simulink model "BMD_2_backup"  (R2025b)
settings: Solver=FixedStepAuto  StartTime=0.0  StopTime=15  FixedStep=0.005  RelTol=1e-3
values from neighbouring files (symbols this model uses):
  FPV_mass = 0.8    [Soft.m]
  g = 9.81    [Soft.m]
  ks = 0    [Soft.m]
  p_0 = 1013.25    [Soft.m]
  Q2Ts = forcetomotors()    [Soft.m]    (also in forcetomotors.m = inv(Ts2Q))
  takeOffDuration = 2    [Soft.m]
  Ts = 0.005    [Soft.m]
undefined symbols (not defined in the file or in its folder): CdA, DiscIntNeverNeededParam, Dw, kd_dz, kd_pos_dx, kd_pos_dy, kd_pq, kd_pr, kd_y, kd_z, ki_dz, ki_pos_dx, ki_pos_dy, ki_pq, ki_pr, ki_y, ki_z, kp_dz, kp_pos_dx, kp_pos_dy, kp_pos_x, kp_pos_y, kp_pq, kp_pr, kp_y, kp_z, pInitialization, rho
libraries: simulink x43, discretizing x18, slpidlib x3, SignalEditorBlockLib x2, shared6dof x1, dynamicsLibrary x1, aerolibasang x1, aerolibnav x1
(part 7 of 22)

== system BMD_2_backup/FCS/Controller/tau_contorller ==
  Yaw_ref [rad/s] : Inport
  In2 : Inport  Port=2
  r_s : Inport  Port=3
  In4 : Inport  Port=4
  Compare To Constant : simulink/Logic and Bit Operations/Compare To Constant  relop===  const=0.00  OutDataTypeStr=boolean
  Constant1 : Constant  Value=0
  Discrete-Time Integrator : DiscreteIntegrator  gainval=0.05  SampleTime=-1  ICPrevOutput=DiscIntNeverNeededParam  ICPrevScaledInput=DiscIntNeverNeededParam
  Gain1 : Gain  Gain=0.8
  Gain_yaw_in : Gain  Gain=1.3
  NOT : Logic  Operator=NOT  IconShape=distinctive  AllPortsSameDT=off  OutDataTypeStr=boolean
  PID Controller (2DOF) : slpidlib/PID Controller (2DOF)  Controller=PID  Form=Parallel  TimeDomain=Discrete-time  UseExternalTs=off  SampleTime=0.005  IntegratorMethod=Forward Euler  FilterMethod=Forward Euler  ControllerParametersSource=internal  P=kp_y  I=ki_y  UseKiTs=off  D=kd_y  UseExternalDerivativeSource=off  N=100  UseFilter=on  b=1  c=0  TunerSelectOption=Transfer Function Based (PID Tuner App)  InitialConditionSource=internal  InitialConditionForIntegrator=0  InitialConditionForFilter=0  DifferentiatorICPrevScaledInput=0  ExternalReset=none  TrackingMode=off  Kt=1  LimitOutput=off  SatLimitsSource=internal  UpperSaturationLimit=inf  LowerSaturationLimit=-inf  LinearizeAsGain=on  AntiWindupMode=none  Kb=1  LimitIntegrator=on  UpperIntegratorSaturationLimit=0.02  LowerIntegratorSaturationLimit=-0.02  POutMin=[]  POutMax=[]  IOutMin=[]  IOutMax=[]  DOutMin=[]  DOutMax=[]  NOutMin=[]  NOutMax=[]  bOutMin=[]  bOutMax=[]  cOutMin=[]  cOutMax=[]  SumOutMin=[]  SumOutMax=[]  SaturationOutMin=[]  SaturationOutMax=[]  PParamMin=[]  PParamMax=[]  IParamMin=[]  IParamMax=[]  DParamMin=[]  DParamMax=[]  NParamMin=[]  NParamMax=[]  bParamMin=[]  bParamMax=[]  cParamMin=[]  cParamMax=[]  KbParamMin=[]  KbParamMax=[]  KtParamMin=[]  KtParamMax=[]  KbOutMin=[]  KbOutMax=[]  KtOutMin=[]  KtOutMax=[]  IntegratorOutMin=[]  IntegratorOutMax=[]  FilterOutMin=[]  FilterOutMax=[]  SumI1OutMin=[]  SumI1OutMax=[]  SumI2OutMin=[]  SumI2OutMax=[]  SumI3OutMin=[]  SumI3OutMax=[]  SumI4OutMin=[]  SumI4OutMax=[]  SumDOutMin=[]  SumDOutMax=[]  Sum1OutMin=[]  Sum1OutMax=[]  Sum2OutMin=[]  Sum2OutMax=[]  Sum3OutMin=[]  Sum3OutMax=[]  DifferentiatorOutMin=[]  DifferentiatorOutMax=[]  FilterDiffOutCoefMin=[]  FilterDiffOutCoefMax=[]  ReciprocalOutMin=[]  ReciprocalOutMax=[]  SumDenOutMin=[]  SumDenOutMax=[]  SumNumOutMin=[]  SumNumOutMax=[]  DivideOutMin=[]  DivideOutMax=[]  UdiffTsProdOutMin=[]  UdiffTsProdOutMax=[]  NTsProdOutMin=[]  NTsProdOutMax=[]  UintegralTsProdOutMin=[]  UintegralTsProdOutMax=[]  UngainTsProdOutMin=[]  UngainTsProdOutMax=[]  ClampingZeroOutDataTypeStr=Inherit: Inherit via back propagation  ClampingZeroOutMin=[]  ClampingZeroOutMax=[]  FilterDenConstantOutDataTypeStr=Inherit: Inherit via back propagation  FilterDenConstantOutMin=[]  FilterDenConstantOutMax=[]  PCopyOutDataTypeStr=Inherit: Inherit via back propagation  PCopyOutMin=[]  PCopyOutMax=[]  NCopyOutDataTypeStr=Inherit: Inherit via back propagation  NCopyOutMin=[]  NCopyOutMax=[]  IntegratorContinuousStateAttributes=''  IntegratorStateMustResolveToSignalObject=off  IntegratorRTWStateStorageClass=Auto  FilterContinuousStateAttributes=''  FilterStateMustResolveToSignalObject=off  FilterRTWStateStorageClass=Auto  ParallelPVariant=InternalParameters  IdealPVariant=Disabled  IVariant=InternalParameters  DVariant=InternalParameters  bVariant=InternalParameters  cVariant=InternalParameters  IntegratorVariant=Discrete  SatVariant=Disabled  AWVariant=Passthrough  PCopyVariant=Disabled  TRVariant=Disabled  FdbkBlocksVariant=Forward  IdealPFdbkVariant=Disabled  SatFdbkVariant=Disabled  DerivativeFilterVariant=ForwardEulerFilter  NVariant=InternalParameters  NCopyVariant=Disabled  FilterICVariant=InternalICsFilter  IntegratorICVariant=InternalICs  ExternalResetVariant=Disabled  TRSumVariant=Passthrough  SumFdbkVariant=Disabled  SumVariant=Sum_PID  TsampFilterVariant=InternalTs  TsampNgainVariant=Passthrough  TsampIntegralVariant=Disabled_SignalSpec  ExternalSaturationOutDataTypeStr=Inherit: Same as second input  DerivativeSourceVariant=ErrorSignal  PreIntVariant=InternalPreInt
  Rate Limiter1 : RateLimiter  RisingSlewLimit=2.0  FallingSlewLimit=-2.0  SampleTimeMode=inherited
  Saturation : Saturate  LinearizeAsGain=off
  Saturation_yaw_out : Saturate  UpperLimit=05  OutDataTypeStr=double
  Scope : Scope
      settings: ActiveDisplayYMinimum=-1  ActiveDisplayYMaximum=1  DataLoggingVariableName=ScopeData36
  Scope2 : Scope
      settings: ActiveDisplayYMinimum=-0.021957566607169628  ActiveDisplayYMaximum=0.19761914569671202  DataLoggingVariableName=ScopeData40
  Sum : Sum  Inputs=|+-
  Sum1 : Sum  Inputs=|++
  Switch1 : Switch  Criteria=u2 > Threshold  OutDataTypeStr=single  SaturateOnIntegerOverflow=off  InputSameDT=off
  Switch2 : Switch  Criteria=u2 > Threshold  OutDataTypeStr=single  SaturateOnIntegerOverflow=off  InputSameDT=off
  Switch3 : Switch  Criteria=u2 > Threshold  OutDataTypeStr=single  SaturateOnIntegerOverflow=off  InputSameDT=off
  Terminator : Terminator
  Unit Delay : UnitDelay  SampleTime=-1  HasFrameUpgradeWarning=on
  tau_yaw : Outport
  wires:
  Discrete-Time Integrator/1 -> Scope/1
  Constant1/1 -> Switch1/1
  Yaw_ref [rad/s]/1 -> Compare To Constant/1, Switch1/3
  Rate Limiter1/1 -> Gain_yaw_in/1
  Saturation_yaw_out/1 -> tau_yaw/1
  Switch1/1 -> Rate Limiter1/1
  In2/1 -> Terminator/1
  PID Controller (2DOF)/1 -> Saturation_yaw_out/1
  Compare To Constant/1 -> Switch2/2, NOT/1, Switch1/2
  In4/1 -> Sum/2, Switch2/3
  Switch2/1 -> Unit Delay/1, Scope2/1, Sum/1
  Unit Delay/1 -> Switch2/1
  Sum/1 -> Gain1/1
  Gain1/1 -> Sum1/2
  Sum1/1 -> Saturation/1
  NOT/1 -> Switch3/2
  Gain_yaw_in/1 -> Switch3/1
  Switch3/1 -> PID Controller (2DOF)/1
  Saturation/1 -> Switch3/3
  r_s/1 -> Discrete-Time Integrator/1, PID Controller (2DOF)/2

== system BMD_2_backup/FCS/filters/Subsystem ==
  GPS_s : Inport
  pressure_f : Inport  Port=2
  ax,ay,ax_f : Inport  Port=3
  orient_earth : Inport  Port=4
  Data Type Conversion3 : DataTypeConversion  OutDataTypeStr=single  SaturateOnIntegerOverflow=off  RndMeth=Floor
  Scope : Scope  NumInputPorts=2
      settings: ActiveDisplayYMinimum=-1.9435508120805021  ActiveDisplayYMaximum=15.792740793898702  DataLoggingVariableName=ScopeData52
  Scope1 : Scope
      settings: ActiveDisplayYMinimum=-1  ActiveDisplayYMaximum=1  DataLoggingVariableName=ScopeData55
  body2earth : Subsystem
  x,y,z,dy,dy,dz : Subsystem
  x,y,z : Outport
  dx,dy,dz : Outport  Port=2
  wires:
  x,y,z,dy,dy,dz/2(dx,dy,dz) -> Scope1/1, dx,dy,dz/1
  body2earth/1(Out1) -> x,y,z,dy,dy,dz/1(ax,ay,az_earth)  "ax,ay,az_earth"
  orient_earth/1 -> Data Type Conversion3/1
  ax,ay,ax_f/1 -> body2earth/1(ax,ay,az)
  x,y,z,dy,dy,dz/1(x,y,z) -> Scope/1, x,y,z/1
  pressure_f/1 -> x,y,z,dy,dy,dz/2(pressure_f)
  Data Type Conversion3/1 -> body2earth/2(orient_f)
  GPS_s/1 -> x,y,z,dy,dy,dz/3(GPS_s)

== system BMD_2_backup/FCS/filters/Subsystem1 ==
  ax,ay,ax_f : Inport
  p,q,r_f : Inport  Port=2
  Demux2 : Demux  Outputs=3
  Mux1 : Mux  Inputs=3
  pitch_kalman : Subsystem
  roll_kalman : Subsystem
  yaw_filter : Subsystem
  orient_earth : Outport
  wires:
  Mux1/1 -> orient_earth/1  "orient_earth"
  Demux2/3 -> yaw_filter/1(In1)  "r"
  Demux2/2 -> pitch_kalman/2(pitch)  "q"
  ax,ay,ax_f/1 -> roll_kalman/1(ax,ay,az), pitch_kalman/1(ax,ay,az)
  Demux2/1 -> roll_kalman/2(p)  "p"
  pitch_kalman/1(Out1) -> Mux1/2  "pitch_f"
  p,q,r_f/1 -> Demux2/1
  yaw_filter/1(Out1) -> Mux1/3  "yaw_f"
  roll_kalman/1(roll_f) -> Mux1/1  "roll_f"

== system BMD_2_backup/FCS/filters/pqr_LPF1 ==
  1 : Inport
  Demux : Demux  Outputs=3
  Mux : Mux  Inputs=3
  Transfer Fcn1 : discretizing/Discretized Transfer Fcn  Numerator=[1]  Denominator=[0.15 1]  AbsTol=auto  SampleTime=0.005  method=zoh  Wc=0
  Transfer Fcn2 : discretizing/Discretized Transfer Fcn  Numerator=[1]  Denominator=[0.15 1]  AbsTol=auto  SampleTime=0.005  method=zoh  Wc=0
  Transfer Fcn3 : discretizing/Discretized Transfer Fcn  Numerator=[1]  Denominator=[0.15 1]  AbsTol=auto  SampleTime=0.005  method=zoh  Wc=0
  ax,ay,az : Outport
  wires:
  1/1 -> Demux/1
  Mux/1 -> ax,ay,az/1
  Demux/1 -> Transfer Fcn3/1
  Demux/2 -> Transfer Fcn1/1
  Demux/3 -> Transfer Fcn2/1
  Transfer Fcn3/1 -> Mux/1
  Transfer Fcn2/1 -> Mux/3
  Transfer Fcn1/1 -> Mux/2

== system BMD_2_backup/FCS/filters/pqr_LPF2 ==
  p,q,r : Inport
  Demux : Demux  Outputs=3
  Mux : Mux  Inputs=3
  Transfer Fcn1 : discretizing/Discretized Transfer Fcn  Numerator=[1]  Denominator=[0.15 1]  AbsTol=auto  SampleTime=0.005  method=zoh  Wc=0
  Transfer Fcn2 : discretizing/Discretized Transfer Fcn  Numerator=[1]  Denominator=[0.15 1]  AbsTol=auto  SampleTime=0.005  method=zoh  Wc=0
  Transfer Fcn3 : discretizing/Discretized Transfer Fcn  Numerator=[1]  Denominator=[0.15 1]  AbsTol=auto  SampleTime=0.005  method=zoh  Wc=0
  p,q,r_f : Outport
  wires:
  p,q,r/1 -> Demux/1
  Mux/1 -> p,q,r_f/1
  Demux/1 -> Transfer Fcn3/1
  Demux/2 -> Transfer Fcn1/1
  Demux/3 -> Transfer Fcn2/1
  Transfer Fcn2/1 -> Mux/3  "temp_f"
  Transfer Fcn3/1 -> Mux/1  "temp_f"
  Transfer Fcn1/1 -> Mux/2  "temp_f"

== system BMD_2_backup/Model/Subsystem/Motor Forces and Torques ==
  Vb : Inport
  Density : Inport  Port=2
  pqr : Inport  Port=3
  Motor Commands : Inport  Port=4
  D1 : Constant  Value=0.044
  D2 : Constant  Value=0.044
  D3 : Constant  Value=-0.044
  D4 : Constant  Value=-0.044
  For Each Subsystem : Subsystem  TreatAsAtomicUnit=on
  Gain : Gain  Gain=[0.0030015 0.0030015 0.0030015 0.0030015]
  MotorsToW : Subsystem
  Sum of Elements : Sum  Inputs=+  CollapseMode=Specified dimension  CollapseDim=2
  Sum of Elements1 : Sum  Inputs=+  CollapseMode=Specified dimension  CollapseDim=2
  Vector Concatenate : Concatenate  NumInputs=4  Mode=Multidimensional array  ConcatenateDimension=2
  Motor Forces : Outport  Unit=N  VectorParamsAs1DForOutWhenUnconnected=off
  Motor Torques : Outport  Port=2  Unit=N*m  VectorParamsAs1DForOutWhenUnconnected=off
  wires:
  D4/1 -> Vector Concatenate/4
  Vector Concatenate/1 -> For Each Subsystem/5(D)
  For Each Subsystem/2(Moments) -> Sum of Elements1/1
  pqr/1 -> For Each Subsystem/3(Omega)
  Vb/1 -> For Each Subsystem/1(Vb)
  D1/1 -> Vector Concatenate/1
  D3/1 -> Vector Concatenate/3
  D2/1 -> Vector Concatenate/2
  Sum of Elements1/1 -> Motor Torques/1
  Density/1 -> For Each Subsystem/2(rho)
  Sum of Elements/1 -> Motor Forces/1
  For Each Subsystem/1(Forces) -> Sum of Elements/1
  Motor Commands/1 -> Gain/1
  Gain/1 -> For Each Subsystem/4(w)

== system BMD_2_backup/Model/Subsystem/drag forces ==
  pressure : Inport
  V_b : Inport  Port=2
  Dynamic Pressure : aerolibasang/Dynamic Pressure
  Out1 : Outport
  wires:
  Dynamic Pressure/1 -> Out1/1
  V_b/1 -> Dynamic Pressure/1
  pressure/1 -> Dynamic Pressure/2

== system BMD_2_backup/Model/Subsystem/gravity forces ==
  gravity : Inport
  DCM(angeles) : Inport  Port=2
  Display : Display
  Gain : Gain  Gain=FPV_mass
  Matrix Multiply : Product  Multiplication=Matrix(*)
  Scope : Scope
      settings: ActiveDisplayYMinimum=-0.613125221623891  ActiveDisplayYMaximum=5.5181252577452655  DataLoggingVariableName=ScopeData70
  Out1 : Outport
  wires:
  gravity/1 -> Gain/1
  Gain/1 -> Matrix Multiply/2
  Matrix Multiply/1 -> Display/1, Scope/1, Out1/1
  DCM(angeles)/1 -> Matrix Multiply/1

== system BMD_2_backup/Sensors/Subsystem/Subsystem ==
  Mux : Mux  Inputs=3
  Zero1 : Constant  Value=0  OutDataTypeStr=single
  Zero2 : Constant  Value=0  OutDataTypeStr=single
  Zero3 : Constant  Value=0  OutDataTypeStr=single
  Out1 : Outport
  wires:
  Zero2/1 -> Mux/1
  Zero1/1 -> Mux/2
  Zero3/1 -> Mux/3
  Mux/1 -> Out1/1

== system BMD_2_backup/Sensors/Subsystem1/Subsystem ==
  Mux : Mux  Inputs=3
  Zero1 : Constant  Value=0  OutDataTypeStr=single
  Zero2 : Constant  Value=0  OutDataTypeStr=single
  Zero3 : Constant  Value=0  OutDataTypeStr=single
  Out1 : Outport
  wires:
  Zero2/1 -> Mux/1
  Zero1/1 -> Mux/2
  Zero3/1 -> Mux/3
  Mux/1 -> Out1/1

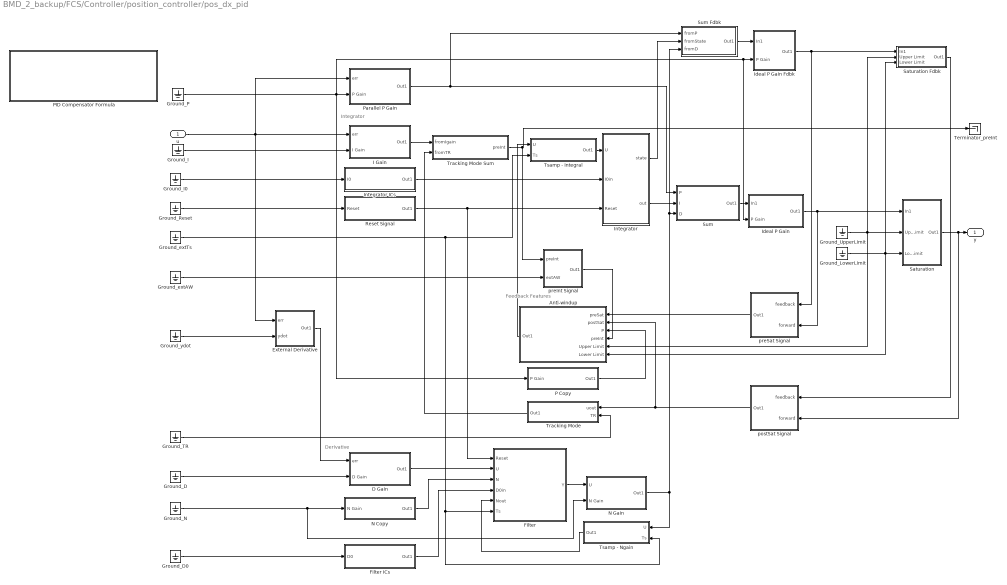
== system BMD_2_backup/FCS/Controller/position_controller/pos_dx_pid ==
  note: Feedback Features
  note: Derivative
  note: Integrator
  u : Inport  SampleTime=SampleTime
  Anti-windup : Subsystem  Variant=on  VariantControlMode=label  VariantControl=Variant1  LabelModeActiveChoice=Passthrough
  D Gain : Subsystem  Variant=on  VariantControlMode=label  VariantControl=Variant1  LabelModeActiveChoice=InternalParameters
  External Derivative : Subsystem  Variant=on  VariantControlMode=label  VariantControl=Variant1  LabelModeActiveChoice=ErrorSignal
  Filter : Subsystem  Variant=on  VariantControlMode=label  LabelModeActiveChoice=ForwardEulerFilter
  Filter ICs : Subsystem  Variant=on  VariantControlMode=label  VariantControl=Variant1  LabelModeActiveChoice=InternalICsFilter
  Ground_D : Ground
  Ground_D0 : Ground
  Ground_I : Ground
  Ground_I0 : Ground
  Ground_LowerLimit : Ground
  Ground_N : Ground
  Ground_P : Ground
  Ground_Reset : Ground
  Ground_TR : Ground  DisableCoverage=on
  Ground_UpperLimit : Ground
  Ground_extAW : Ground
  Ground_extTs : Ground
  Ground_ydot : Ground
  I Gain : Subsystem  Variant=on  VariantControlMode=label  VariantControl=Variant1  LabelModeActiveChoice=InternalParameters
  Ideal P Gain : Subsystem  Variant=on  VariantControlMode=label  VariantControl=Variant1  LabelModeActiveChoice=Disabled
  Ideal P Gain Fdbk : Subsystem  Variant=on  VariantControlMode=label  VariantControl=Variant1  LabelModeActiveChoice=Disabled
  Integrator : Subsystem  Variant=on  VariantControlMode=label  LabelModeActiveChoice=Discrete
  Integrator ICs : Subsystem  Variant=on  VariantControlMode=label  VariantControl=Variant1  LabelModeActiveChoice=InternalICs
  N Copy : Subsystem  Variant=on  VariantControlMode=label  LabelModeActiveChoice=Disabled
  N Gain : Subsystem  Variant=on  VariantControlMode=label  VariantControl=Variant1  LabelModeActiveChoice=InternalParameters
  P Copy : Subsystem  Variant=on  VariantControlMode=label  LabelModeActiveChoice=Disabled
  PID Compensator Formula : Subsystem
      mask Display: image('C:\Program Files\MATLAB\R2025b\toolbox\simulink\library\pid\pid_Images\PID_Parallel_DT_00.png','center');
  Parallel P Gain : Subsystem  Variant=on  VariantControlMode=label  VariantControl=Variant1  LabelModeActiveChoice=InternalParameters
  Reset Signal : Subsystem  Variant=on  VariantControlMode=label  VariantControl=Variant1  LabelModeActiveChoice=Disabled
  Saturation : Subsystem  Variant=on  VariantControlMode=label  LabelModeActiveChoice=Enabled
  Saturation Fdbk : Subsystem  Variant=on  VariantControlMode=label  LabelModeActiveChoice=Disabled
  Sum : Subsystem  Variant=on  VariantControlMode=label  LabelModeActiveChoice=Sum_PID
  Sum Fdbk : Subsystem  DisableCoverage=on  Variant=on  VariantControlMode=label  LabelModeActiveChoice=Disabled
  Terminator_preInt : Terminator
  Tracking Mode : Subsystem  Variant=on  VariantControlMode=label  VariantControl=Variant1  LabelModeActiveChoice=Disabled
  Tracking Mode Sum : Subsystem  Variant=on  VariantControlMode=label  LabelModeActiveChoice=Passthrough
  Tsamp - Integral : Subsystem  Variant=on  VariantControlMode=label  LabelModeActiveChoice=Disabled_SignalSpec
  Tsamp - Ngain : Subsystem  Variant=on  VariantControlMode=label  LabelModeActiveChoice=Passthrough
  postSat Signal : Subsystem  Variant=on  VariantControlMode=label  VariantControl=Variant1  LabelModeActiveChoice=Forward
  preInt Signal : Subsystem  Variant=on  VariantControlMode=label  VariantControl=Variant1  LabelModeActiveChoice=InternalPreInt
  preSat Signal : Subsystem  Variant=on  VariantControlMode=label  VariantControl=Variant1  LabelModeActiveChoice=Forward
  y : Outport  SampleTime=SampleTime
  wires:
  Ground_extAW/1 -> preInt Signal/2(extAW)
  preInt Signal/1(Out1) -> Anti-windup/4(preInt)
  External Derivative/1(Out1) -> D Gain/1(err)
  Ground_ydot/1 -> External Derivative/2(ydot)
  Ground_LowerLimit/1 -> Saturation/3(Lower Limit), Anti-windup/6(Lower Limit), Saturation Fdbk/3(Lower Limit)
  Ground_UpperLimit/1 -> Saturation/2(Upper Limit), Saturation Fdbk/2(Upper Limit), Anti-windup/5(Upper Limit)
  Tsamp - Ngain/1(Out1) -> Filter/5(Nout)
  Anti-windup/1(Out1) -> Tsamp - Integral/1(U)
  Ground_extTs/1 -> Tsamp - Integral/2(Ts), Filter/6(Ts), Tsamp - Ngain/2(Ts)
  Tsamp - Integral/1(Out1) -> Integrator/1(U)
  Tracking Mode/1(Out1) -> Tracking Mode Sum/2(fromTR)
  Ground_I0/1 -> Integrator ICs/1(I0)
  Filter ICs/1(Out1) -> Filter/4(D0in)
  N Copy/1(Out1) -> Filter/3(N)
  D Gain/1(Out1) -> Filter/2(U)
  Ground_D0/1 -> Filter ICs/1(D0)
  Ground_Reset/1 -> Reset Signal/1(Reset)
  N Gain/1(Out1) -> Tsamp - Ngain/1(U), Sum/3(D), Sum Fdbk/3(fromD)
  postSat Signal/1(Out1) -> Anti-windup/2(postSat), Tracking Mode/1(uout)
  preSat Signal/1(Out1) -> Anti-windup/1(preSat)
  Saturation Fdbk/1(Out1) -> postSat Signal/1(feedback)
  P Copy/1(Out1) -> Anti-windup/3(P)
  Ground_TR/1 -> Tracking Mode/2(TR)
  Ground_N/1 -> N Copy/1(N Gain), N Gain/2(N Gain)
  Ideal P Gain Fdbk/1(Out1) -> preSat Signal/1(feedback), Saturation Fdbk/1(In1)
  Sum Fdbk/1(Out1) -> Ideal P Gain Fdbk/1(In1)
  I Gain/1(Out1) -> Tracking Mode Sum/1(fromIgain)
  Saturation/1(Out1) -> y/1, postSat Signal/2(forward)
  Filter/1(Y) -> N Gain/1(U)
  Ground_D/1 -> D Gain/2(D Gain)
  Ideal P Gain/1(Out1) -> Saturation/1(In1), preSat Signal/2(forward)
  u/1 -> External Derivative/1(err), Parallel P Gain/1(err), I Gain/1(err)
  Parallel P Gain/1(Out1) -> Sum/1(P), Sum Fdbk/1(fromP)
  Sum/1(Out1) -> Ideal P Gain/1(In1)
  Ground_P/1 -> Ideal P Gain Fdbk/2(P Gain), Ideal P Gain/2(P Gain), Parallel P Gain/2(P Gain), P Copy/1(P Gain)
  Tracking Mode Sum/1(preInt) -> Terminator_preInt/1, preInt Signal/1(preInt)
  Ground_I/1 -> I Gain/2(I Gain)
  Integrator ICs/1(Out1) -> Integrator/2(I0in)
  Integrator/2(out) -> Sum/2(I)
  Integrator/1(state) -> Sum Fdbk/2(fromState)
  Reset Signal/1(Out1) -> Filter/1(Reset), Integrator/3(Reset)

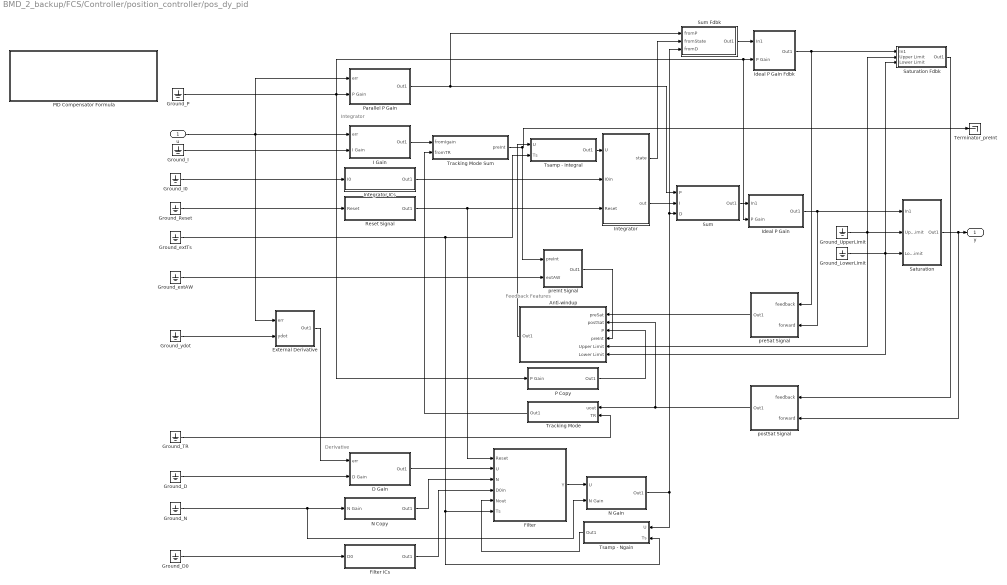
== system BMD_2_backup/FCS/Controller/position_controller/pos_dy_pid ==
  note: Feedback Features
  note: Derivative
  note: Integrator
  u : Inport  SampleTime=SampleTime
  Anti-windup : Subsystem  Variant=on  VariantControlMode=label  VariantControl=Variant1  LabelModeActiveChoice=Passthrough
  D Gain : Subsystem  Variant=on  VariantControlMode=label  VariantControl=Variant1  LabelModeActiveChoice=InternalParameters
  External Derivative : Subsystem  Variant=on  VariantControlMode=label  VariantControl=Variant1  LabelModeActiveChoice=ErrorSignal
  Filter : Subsystem  Variant=on  VariantControlMode=label  LabelModeActiveChoice=ForwardEulerFilter
  Filter ICs : Subsystem  Variant=on  VariantControlMode=label  VariantControl=Variant1  LabelModeActiveChoice=InternalICsFilter
  Ground_D : Ground
  Ground_D0 : Ground
  Ground_I : Ground
  Ground_I0 : Ground
  Ground_LowerLimit : Ground
  Ground_N : Ground
  Ground_P : Ground
  Ground_Reset : Ground
  Ground_TR : Ground  DisableCoverage=on
  Ground_UpperLimit : Ground
  Ground_extAW : Ground
  Ground_extTs : Ground
  Ground_ydot : Ground
  I Gain : Subsystem  Variant=on  VariantControlMode=label  VariantControl=Variant1  LabelModeActiveChoice=InternalParameters
  Ideal P Gain : Subsystem  Variant=on  VariantControlMode=label  VariantControl=Variant1  LabelModeActiveChoice=Disabled
  Ideal P Gain Fdbk : Subsystem  Variant=on  VariantControlMode=label  VariantControl=Variant1  LabelModeActiveChoice=Disabled
  Integrator : Subsystem  Variant=on  VariantControlMode=label  LabelModeActiveChoice=Discrete
  Integrator ICs : Subsystem  Variant=on  VariantControlMode=label  VariantControl=Variant1  LabelModeActiveChoice=InternalICs
  N Copy : Subsystem  Variant=on  VariantControlMode=label  LabelModeActiveChoice=Disabled
  N Gain : Subsystem  Variant=on  VariantControlMode=label  VariantControl=Variant1  LabelModeActiveChoice=InternalParameters
  P Copy : Subsystem  Variant=on  VariantControlMode=label  LabelModeActiveChoice=Disabled
  PID Compensator Formula : Subsystem
      mask Display: image('C:\Program Files\MATLAB\R2025b\toolbox\simulink\library\pid\pid_Images\PID_Parallel_DT_00.png','center');
  Parallel P Gain : Subsystem  Variant=on  VariantControlMode=label  VariantControl=Variant1  LabelModeActiveChoice=InternalParameters
  Reset Signal : Subsystem  Variant=on  VariantControlMode=label  VariantControl=Variant1  LabelModeActiveChoice=Disabled
  Saturation : Subsystem  Variant=on  VariantControlMode=label  LabelModeActiveChoice=Enabled
  Saturation Fdbk : Subsystem  Variant=on  VariantControlMode=label  LabelModeActiveChoice=Disabled
  Sum : Subsystem  Variant=on  VariantControlMode=label  LabelModeActiveChoice=Sum_PID
  Sum Fdbk : Subsystem  DisableCoverage=on  Variant=on  VariantControlMode=label  LabelModeActiveChoice=Disabled
  Terminator_preInt : Terminator
  Tracking Mode : Subsystem  Variant=on  VariantControlMode=label  VariantControl=Variant1  LabelModeActiveChoice=Disabled
  Tracking Mode Sum : Subsystem  Variant=on  VariantControlMode=label  LabelModeActiveChoice=Passthrough
  Tsamp - Integral : Subsystem  Variant=on  VariantControlMode=label  LabelModeActiveChoice=Disabled_SignalSpec
  Tsamp - Ngain : Subsystem  Variant=on  VariantControlMode=label  LabelModeActiveChoice=Passthrough
  postSat Signal : Subsystem  Variant=on  VariantControlMode=label  VariantControl=Variant1  LabelModeActiveChoice=Forward
  preInt Signal : Subsystem  Variant=on  VariantControlMode=label  VariantControl=Variant1  LabelModeActiveChoice=InternalPreInt
  preSat Signal : Subsystem  Variant=on  VariantControlMode=label  VariantControl=Variant1  LabelModeActiveChoice=Forward
  y : Outport  SampleTime=SampleTime
  wires:
  Ground_extAW/1 -> preInt Signal/2(extAW)
  preInt Signal/1(Out1) -> Anti-windup/4(preInt)
  External Derivative/1(Out1) -> D Gain/1(err)
  Ground_ydot/1 -> External Derivative/2(ydot)
  Ground_LowerLimit/1 -> Saturation/3(Lower Limit), Anti-windup/6(Lower Limit), Saturation Fdbk/3(Lower Limit)
  Ground_UpperLimit/1 -> Saturation/2(Upper Limit), Saturation Fdbk/2(Upper Limit), Anti-windup/5(Upper Limit)
  Tsamp - Ngain/1(Out1) -> Filter/5(Nout)
  Anti-windup/1(Out1) -> Tsamp - Integral/1(U)
  Ground_extTs/1 -> Tsamp - Integral/2(Ts), Filter/6(Ts), Tsamp - Ngain/2(Ts)
  Tsamp - Integral/1(Out1) -> Integrator/1(U)
  Tracking Mode/1(Out1) -> Tracking Mode Sum/2(fromTR)
  Ground_I0/1 -> Integrator ICs/1(I0)
  Filter ICs/1(Out1) -> Filter/4(D0in)
  N Copy/1(Out1) -> Filter/3(N)
  D Gain/1(Out1) -> Filter/2(U)
  Ground_D0/1 -> Filter ICs/1(D0)
  Ground_Reset/1 -> Reset Signal/1(Reset)
  N Gain/1(Out1) -> Tsamp - Ngain/1(U), Sum/3(D), Sum Fdbk/3(fromD)
  postSat Signal/1(Out1) -> Anti-windup/2(postSat), Tracking Mode/1(uout)
  preSat Signal/1(Out1) -> Anti-windup/1(preSat)
  Saturation Fdbk/1(Out1) -> postSat Signal/1(feedback)
  P Copy/1(Out1) -> Anti-windup/3(P)
  Ground_TR/1 -> Tracking Mode/2(TR)
  Ground_N/1 -> N Copy/1(N Gain), N Gain/2(N Gain)
  Ideal P Gain Fdbk/1(Out1) -> preSat Signal/1(feedback), Saturation Fdbk/1(In1)
  Sum Fdbk/1(Out1) -> Ideal P Gain Fdbk/1(In1)
  I Gain/1(Out1) -> Tracking Mode Sum/1(fromIgain)
  Saturation/1(Out1) -> y/1, postSat Signal/2(forward)
  Filter/1(Y) -> N Gain/1(U)
  Ground_D/1 -> D Gain/2(D Gain)
  Ideal P Gain/1(Out1) -> Saturation/1(In1), preSat Signal/2(forward)
  u/1 -> External Derivative/1(err), Parallel P Gain/1(err), I Gain/1(err)
  Parallel P Gain/1(Out1) -> Sum/1(P), Sum Fdbk/1(fromP)
  Sum/1(Out1) -> Ideal P Gain/1(In1)
  Ground_P/1 -> Ideal P Gain Fdbk/2(P Gain), Ideal P Gain/2(P Gain), Parallel P Gain/2(P Gain), P Copy/1(P Gain)
  Tracking Mode Sum/1(preInt) -> Terminator_preInt/1, preInt Signal/1(preInt)
  Ground_I/1 -> I Gain/2(I Gain)
  Integrator ICs/1(Out1) -> Integrator/2(I0in)
  Integrator/2(out) -> Sum/2(I)
  Integrator/1(state) -> Sum Fdbk/2(fromState)
  Reset Signal/1(Out1) -> Filter/1(Reset), Integrator/3(Reset)

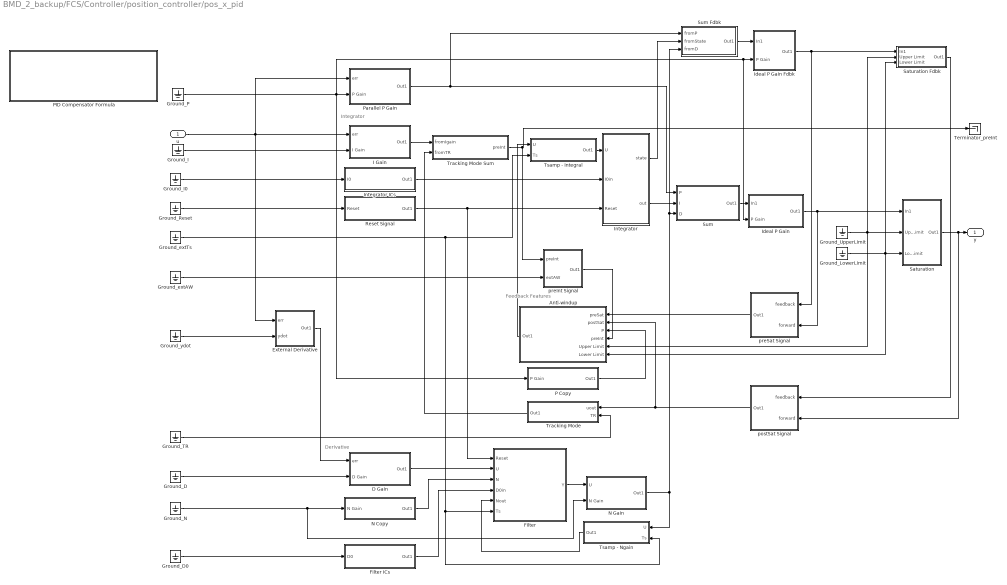
== system BMD_2_backup/FCS/Controller/position_controller/pos_x_pid ==
  note: Feedback Features
  note: Derivative
  note: Integrator
  u : Inport  SampleTime=SampleTime
  Anti-windup : Subsystem  Variant=on  VariantControlMode=label  VariantControl=Variant1  LabelModeActiveChoice=Disabled
  D Gain : Subsystem  Variant=on  VariantControlMode=label  VariantControl=Variant1  LabelModeActiveChoice=Disabled
  External Derivative : Subsystem  Variant=on  VariantControlMode=label  VariantControl=Variant1  LabelModeActiveChoice=Disabled
  Filter : Subsystem  Variant=on  VariantControlMode=label  LabelModeActiveChoice=Disabled
  Filter ICs : Subsystem  Variant=on  VariantControlMode=label  VariantControl=Variant1  LabelModeActiveChoice=Disabled
  Ground_D : Ground
  Ground_D0 : Ground
  Ground_I : Ground
  Ground_I0 : Ground
  Ground_LowerLimit : Ground
  Ground_N : Ground
  Ground_P : Ground
  Ground_Reset : Ground
  Ground_TR : Ground  DisableCoverage=on
  Ground_UpperLimit : Ground
  Ground_extAW : Ground
  Ground_extTs : Ground
  Ground_ydot : Ground
  I Gain : Subsystem  Variant=on  VariantControlMode=label  VariantControl=Variant1  LabelModeActiveChoice=Disabled
  Ideal P Gain : Subsystem  Variant=on  VariantControlMode=label  VariantControl=Variant1  LabelModeActiveChoice=Disabled
  Ideal P Gain Fdbk : Subsystem  Variant=on  VariantControlMode=label  VariantControl=Variant1  LabelModeActiveChoice=Disabled
  Integrator : Subsystem  Variant=on  VariantControlMode=label  LabelModeActiveChoice=Disabled
  Integrator ICs : Subsystem  Variant=on  VariantControlMode=label  VariantControl=Variant1  LabelModeActiveChoice=Disabled
  N Copy : Subsystem  Variant=on  VariantControlMode=label  LabelModeActiveChoice=Disabled_SignalSpec
  N Gain : Subsystem  Variant=on  VariantControlMode=label  VariantControl=Variant1  LabelModeActiveChoice=Disabled
  P Copy : Subsystem  Variant=on  VariantControlMode=label  LabelModeActiveChoice=Disabled
  PID Compensator Formula : Subsystem
      mask Display: image('C:\Program Files\MATLAB\R2025b\toolbox\simulink\library\pid\pid_Images\P.png','center');
  Parallel P Gain : Subsystem  Variant=on  VariantControlMode=label  VariantControl=Variant1  LabelModeActiveChoice=InternalParameters
  Reset Signal : Subsystem  Variant=on  VariantControlMode=label  VariantControl=Variant1  LabelModeActiveChoice=Disabled
  Saturation : Subsystem  Variant=on  VariantControlMode=label  LabelModeActiveChoice=Enabled
  Saturation Fdbk : Subsystem  Variant=on  VariantControlMode=label  LabelModeActiveChoice=Disabled
  Sum : Subsystem  Variant=on  VariantControlMode=label  LabelModeActiveChoice=Passthrough_P
  Sum Fdbk : Subsystem  DisableCoverage=on  Variant=on  VariantControlMode=label  LabelModeActiveChoice=Disabled
  Terminator_preInt : Terminator
  Tracking Mode : Subsystem  Variant=on  VariantControlMode=label  VariantControl=Variant1  LabelModeActiveChoice=Disabled
  Tracking Mode Sum : Subsystem  Variant=on  VariantControlMode=label  LabelModeActiveChoice=Passthrough
  Tsamp - Integral : Subsystem  Variant=on  VariantControlMode=label  LabelModeActiveChoice=Disabled_SignalSpec
  Tsamp - Ngain : Subsystem  Variant=on  VariantControlMode=label  LabelModeActiveChoice=Passthrough
  postSat Signal : Subsystem  Variant=on  VariantControlMode=label  VariantControl=Variant1  LabelModeActiveChoice=Forward
  preInt Signal : Subsystem  Variant=on  VariantControlMode=label  VariantControl=Variant1  LabelModeActiveChoice=InternalPreInt
  preSat Signal : Subsystem  Variant=on  VariantControlMode=label  VariantControl=Variant1  LabelModeActiveChoice=Forward
  y : Outport  SampleTime=SampleTime
  wires:
  Ground_extAW/1 -> preInt Signal/2(extAW)
  preInt Signal/1(Out1) -> Anti-windup/4(preInt)
  External Derivative/1(Out1) -> D Gain/1(err)
  Ground_ydot/1 -> External Derivative/2(ydot)
  Ground_LowerLimit/1 -> Saturation/3(Lower Limit), Anti-windup/6(Lower Limit), Saturation Fdbk/3(Lower Limit)
  Ground_UpperLimit/1 -> Saturation/2(Upper Limit), Saturation Fdbk/2(Upper Limit), Anti-windup/5(Upper Limit)
  Tsamp - Ngain/1(Out1) -> Filter/5(Nout)
  Anti-windup/1(Out1) -> Tsamp - Integral/1(U)
  Ground_extTs/1 -> Tsamp - Integral/2(Ts), Filter/6(Ts), Tsamp - Ngain/2(Ts)
  Tsamp - Integral/1(Out1) -> Integrator/1(U)
  Tracking Mode/1(Out1) -> Tracking Mode Sum/2(fromTR)
  Ground_I0/1 -> Integrator ICs/1(I0)
  Filter ICs/1(Out1) -> Filter/4(D0in)
  N Copy/1(Out1) -> Filter/3(N)
  D Gain/1(Out1) -> Filter/2(U)
  Ground_D0/1 -> Filter ICs/1(D0)
  Ground_Reset/1 -> Reset Signal/1(Reset)
  N Gain/1(Out1) -> Tsamp - Ngain/1(U), Sum/3(D), Sum Fdbk/3(fromD)
  postSat Signal/1(Out1) -> Anti-windup/2(postSat), Tracking Mode/1(uout)
  preSat Signal/1(Out1) -> Anti-windup/1(preSat)
  Saturation Fdbk/1(Out1) -> postSat Signal/1(feedback)
  P Copy/1(Out1) -> Anti-windup/3(P)
  Ground_TR/1 -> Tracking Mode/2(TR)
  Ground_N/1 -> N Copy/1(N Gain), N Gain/2(N Gain)
  Ideal P Gain Fdbk/1(Out1) -> preSat Signal/1(feedback), Saturation Fdbk/1(In1)
  Sum Fdbk/1(Out1) -> Ideal P Gain Fdbk/1(In1)
  I Gain/1(Out1) -> Tracking Mode Sum/1(fromIgain)
  Saturation/1(Out1) -> y/1, postSat Signal/2(forward)
  Filter/1(Y) -> N Gain/1(U)
  Ground_D/1 -> D Gain/2(D Gain)
  Ideal P Gain/1(Out1) -> Saturation/1(In1), preSat Signal/2(forward)
  u/1 -> External Derivative/1(err), Parallel P Gain/1(err), I Gain/1(err)
  Parallel P Gain/1(Out1) -> Sum/1(P), Sum Fdbk/1(fromP)
  Sum/1(Out1) -> Ideal P Gain/1(In1)
  Ground_P/1 -> Ideal P Gain Fdbk/2(P Gain), Ideal P Gain/2(P Gain), Parallel P Gain/2(P Gain), P Copy/1(P Gain)
  Tracking Mode Sum/1(preInt) -> Terminator_preInt/1, preInt Signal/1(preInt)
  Ground_I/1 -> I Gain/2(I Gain)
  Integrator ICs/1(Out1) -> Integrator/2(I0in)
  Integrator/2(out) -> Sum/2(I)
  Integrator/1(state) -> Sum Fdbk/2(fromState)
  Reset Signal/1(Out1) -> Filter/1(Reset), Integrator/3(Reset)

== system BMD_2_backup/FCS/Controller/position_controller/pos_y_pid ==
  note: Feedback Features
  note: Derivative
  note: Integrator
  u : Inport  SampleTime=SampleTime
  Anti-windup : Subsystem  Variant=on  VariantControlMode=label  VariantControl=Variant1  LabelModeActiveChoice=Disabled
  D Gain : Subsystem  Variant=on  VariantControlMode=label  VariantControl=Variant1  LabelModeActiveChoice=Disabled
  External Derivative : Subsystem  Variant=on  VariantControlMode=label  VariantControl=Variant1  LabelModeActiveChoice=Disabled
  Filter : Subsystem  Variant=on  VariantControlMode=label  LabelModeActiveChoice=Disabled
  Filter ICs : Subsystem  Variant=on  VariantControlMode=label  VariantControl=Variant1  LabelModeActiveChoice=Disabled
  Ground_D : Ground
  Ground_D0 : Ground
  Ground_I : Ground
  Ground_I0 : Ground
  Ground_LowerLimit : Ground
  Ground_N : Ground
  Ground_P : Ground
  Ground_Reset : Ground
  Ground_TR : Ground  DisableCoverage=on
  Ground_UpperLimit : Ground
  Ground_extAW : Ground
  Ground_extTs : Ground
  Ground_ydot : Ground
  I Gain : Subsystem  Variant=on  VariantControlMode=label  VariantControl=Variant1  LabelModeActiveChoice=Disabled
  Ideal P Gain : Subsystem  Variant=on  VariantControlMode=label  VariantControl=Variant1  LabelModeActiveChoice=Disabled
  Ideal P Gain Fdbk : Subsystem  Variant=on  VariantControlMode=label  VariantControl=Variant1  LabelModeActiveChoice=Disabled
  Integrator : Subsystem  Variant=on  VariantControlMode=label  LabelModeActiveChoice=Disabled
  Integrator ICs : Subsystem  Variant=on  VariantControlMode=label  VariantControl=Variant1  LabelModeActiveChoice=Disabled
  N Copy : Subsystem  Variant=on  VariantControlMode=label  LabelModeActiveChoice=Disabled_SignalSpec
  N Gain : Subsystem  Variant=on  VariantControlMode=label  VariantControl=Variant1  LabelModeActiveChoice=Disabled
  P Copy : Subsystem  Variant=on  VariantControlMode=label  LabelModeActiveChoice=Disabled
  PID Compensator Formula : Subsystem
      mask Display: image('C:\Program Files\MATLAB\R2025b\toolbox\simulink\library\pid\pid_Images\P.png','center');
  Parallel P Gain : Subsystem  Variant=on  VariantControlMode=label  VariantControl=Variant1  LabelModeActiveChoice=InternalParameters
  Reset Signal : Subsystem  Variant=on  VariantControlMode=label  VariantControl=Variant1  LabelModeActiveChoice=Disabled
  Saturation : Subsystem  Variant=on  VariantControlMode=label  LabelModeActiveChoice=Enabled
  Saturation Fdbk : Subsystem  Variant=on  VariantControlMode=label  LabelModeActiveChoice=Disabled
  Sum : Subsystem  Variant=on  VariantControlMode=label  LabelModeActiveChoice=Passthrough_P
  Sum Fdbk : Subsystem  DisableCoverage=on  Variant=on  VariantControlMode=label  LabelModeActiveChoice=Disabled
  Terminator_preInt : Terminator
  Tracking Mode : Subsystem  Variant=on  VariantControlMode=label  VariantControl=Variant1  LabelModeActiveChoice=Disabled
  Tracking Mode Sum : Subsystem  Variant=on  VariantControlMode=label  LabelModeActiveChoice=Passthrough
  Tsamp - Integral : Subsystem  Variant=on  VariantControlMode=label  LabelModeActiveChoice=Disabled_SignalSpec
  Tsamp - Ngain : Subsystem  Variant=on  VariantControlMode=label  LabelModeActiveChoice=Passthrough
  postSat Signal : Subsystem  Variant=on  VariantControlMode=label  VariantControl=Variant1  LabelModeActiveChoice=Forward
  preInt Signal : Subsystem  Variant=on  VariantControlMode=label  VariantControl=Variant1  LabelModeActiveChoice=InternalPreInt
  preSat Signal : Subsystem  Variant=on  VariantControlMode=label  VariantControl=Variant1  LabelModeActiveChoice=Forward
  y : Outport  SampleTime=SampleTime
  wires:
  Ground_extAW/1 -> preInt Signal/2(extAW)
  preInt Signal/1(Out1) -> Anti-windup/4(preInt)
  External Derivative/1(Out1) -> D Gain/1(err)
  Ground_ydot/1 -> External Derivative/2(ydot)
  Ground_LowerLimit/1 -> Saturation/3(Lower Limit), Anti-windup/6(Lower Limit), Saturation Fdbk/3(Lower Limit)
  Ground_UpperLimit/1 -> Saturation/2(Upper Limit), Saturation Fdbk/2(Upper Limit), Anti-windup/5(Upper Limit)
  Tsamp - Ngain/1(Out1) -> Filter/5(Nout)
  Anti-windup/1(Out1) -> Tsamp - Integral/1(U)
  Ground_extTs/1 -> Tsamp - Integral/2(Ts), Filter/6(Ts), Tsamp - Ngain/2(Ts)
  Tsamp - Integral/1(Out1) -> Integrator/1(U)
  Tracking Mode/1(Out1) -> Tracking Mode Sum/2(fromTR)
  Ground_I0/1 -> Integrator ICs/1(I0)
  Filter ICs/1(Out1) -> Filter/4(D0in)
  N Copy/1(Out1) -> Filter/3(N)
  D Gain/1(Out1) -> Filter/2(U)
  Ground_D0/1 -> Filter ICs/1(D0)
  Ground_Reset/1 -> Reset Signal/1(Reset)
  N Gain/1(Out1) -> Tsamp - Ngain/1(U), Sum/3(D), Sum Fdbk/3(fromD)
  postSat Signal/1(Out1) -> Anti-windup/2(postSat), Tracking Mode/1(uout)
  preSat Signal/1(Out1) -> Anti-windup/1(preSat)
  Saturation Fdbk/1(Out1) -> postSat Signal/1(feedback)
  P Copy/1(Out1) -> Anti-windup/3(P)
  Ground_TR/1 -> Tracking Mode/2(TR)
  Ground_N/1 -> N Copy/1(N Gain), N Gain/2(N Gain)
  Ideal P Gain Fdbk/1(Out1) -> preSat Signal/1(feedback), Saturation Fdbk/1(In1)
  Sum Fdbk/1(Out1) -> Ideal P Gain Fdbk/1(In1)
  I Gain/1(Out1) -> Tracking Mode Sum/1(fromIgain)
  Saturation/1(Out1) -> y/1, postSat Signal/2(forward)
  Filter/1(Y) -> N Gain/1(U)
  Ground_D/1 -> D Gain/2(D Gain)
  Ideal P Gain/1(Out1) -> Saturation/1(In1), preSat Signal/2(forward)
  u/1 -> External Derivative/1(err), Parallel P Gain/1(err), I Gain/1(err)
  Parallel P Gain/1(Out1) -> Sum/1(P), Sum Fdbk/1(fromP)
  Sum/1(Out1) -> Ideal P Gain/1(In1)
  Ground_P/1 -> Ideal P Gain Fdbk/2(P Gain), Ideal P Gain/2(P Gain), Parallel P Gain/2(P Gain), P Copy/1(P Gain)
  Tracking Mode Sum/1(preInt) -> Terminator_preInt/1, preInt Signal/1(preInt)
  Ground_I/1 -> I Gain/2(I Gain)
  Integrator ICs/1(Out1) -> Integrator/2(I0in)
  Integrator/2(out) -> Sum/2(I)
  Integrator/1(state) -> Sum Fdbk/2(fromState)
  Reset Signal/1(Out1) -> Filter/1(Reset), Integrator/3(Reset)

== system BMD_2_backup/FCS/Controller/roll_pitch_controller/PID Controller ==
  note: Feedback Features
  note: Derivative
  note: Integrator
  u : Inport  SampleTime=SampleTime
  Anti-windup : Subsystem  Variant=on  VariantControlMode=label  VariantControl=Variant1  LabelModeActiveChoice=Passthrough
  D Gain : Subsystem  Variant=on  VariantControlMode=label  VariantControl=Variant1  LabelModeActiveChoice=InternalParameters
  External Derivative : Subsystem  Variant=on  VariantControlMode=label  VariantControl=Variant1  LabelModeActiveChoice=ErrorSignal
  Filter : Subsystem  Variant=on  VariantControlMode=label  LabelModeActiveChoice=ForwardEulerFilter
  Filter ICs : Subsystem  Variant=on  VariantControlMode=label  VariantControl=Variant1  LabelModeActiveChoice=InternalICsFilter
  Ground_D : Ground
  Ground_D0 : Ground
  Ground_I : Ground
  Ground_I0 : Ground
  Ground_LowerLimit : Ground
  Ground_N : Ground
  Ground_P : Ground
  Ground_Reset : Ground
  Ground_TR : Ground  DisableCoverage=on
  Ground_UpperLimit : Ground
  Ground_extAW : Ground
  Ground_extTs : Ground
  Ground_ydot : Ground
  I Gain : Subsystem  Variant=on  VariantControlMode=label  VariantControl=Variant1  LabelModeActiveChoice=InternalParameters
  Ideal P Gain : Subsystem  Variant=on  VariantControlMode=label  VariantControl=Variant1  LabelModeActiveChoice=Disabled
  Ideal P Gain Fdbk : Subsystem  Variant=on  VariantControlMode=label  VariantControl=Variant1  LabelModeActiveChoice=Disabled
  Integrator : Subsystem  Variant=on  VariantControlMode=label  LabelModeActiveChoice=Discrete
  Integrator ICs : Subsystem  Variant=on  VariantControlMode=label  VariantControl=Variant1  LabelModeActiveChoice=InternalICs
  N Copy : Subsystem  Variant=on  VariantControlMode=label  LabelModeActiveChoice=Disabled
  N Gain : Subsystem  Variant=on  VariantControlMode=label  VariantControl=Variant1  LabelModeActiveChoice=InternalParameters
  P Copy : Subsystem  Variant=on  VariantControlMode=label  LabelModeActiveChoice=Disabled
  PID Compensator Formula : Subsystem
      mask Display: image('C:\Program Files\MATLAB\R2025b\toolbox\simulink\library\pid\pid_Images\PID_Parallel_DT_00.png','center');
  Parallel P Gain : Subsystem  Variant=on  VariantControlMode=label  VariantControl=Variant1  LabelModeActiveChoice=InternalParameters
  Reset Signal : Subsystem  Variant=on  VariantControlMode=label  VariantControl=Variant1  LabelModeActiveChoice=Disabled
  Saturation : Subsystem  Variant=on  VariantControlMode=label  LabelModeActiveChoice=Disabled
  Saturation Fdbk : Subsystem  Variant=on  VariantControlMode=label  LabelModeActiveChoice=Disabled
  Sum : Subsystem  Variant=on  VariantControlMode=label  LabelModeActiveChoice=Sum_PID
  Sum Fdbk : Subsystem  DisableCoverage=on  Variant=on  VariantControlMode=label  LabelModeActiveChoice=Disabled
  Terminator_preInt : Terminator
  Tracking Mode : Subsystem  Variant=on  VariantControlMode=label  VariantControl=Variant1  LabelModeActiveChoice=Disabled
  Tracking Mode Sum : Subsystem  Variant=on  VariantControlMode=label  LabelModeActiveChoice=Passthrough
  Tsamp - Integral : Subsystem  Variant=on  VariantControlMode=label  LabelModeActiveChoice=Disabled_SignalSpec
  Tsamp - Ngain : Subsystem  Variant=on  VariantControlMode=label  LabelModeActiveChoice=Passthrough
  postSat Signal : Subsystem  Variant=on  VariantControlMode=label  VariantControl=Variant1  LabelModeActiveChoice=Forward
  preInt Signal : Subsystem  Variant=on  VariantControlMode=label  VariantControl=Variant1  LabelModeActiveChoice=InternalPreInt
  preSat Signal : Subsystem  Variant=on  VariantControlMode=label  VariantControl=Variant1  LabelModeActiveChoice=Forward
  y : Outport  SampleTime=SampleTime
  wires:
  Ground_extAW/1 -> preInt Signal/2(extAW)
  preInt Signal/1(Out1) -> Anti-windup/4(preInt)
  External Derivative/1(Out1) -> D Gain/1(err)
  Ground_ydot/1 -> External Derivative/2(ydot)
  Ground_LowerLimit/1 -> Saturation/3(Lower Limit), Anti-windup/6(Lower Limit), Saturation Fdbk/3(Lower Limit)
  Ground_UpperLimit/1 -> Saturation/2(Upper Limit), Saturation Fdbk/2(Upper Limit), Anti-windup/5(Upper Limit)
  Tsamp - Ngain/1(Out1) -> Filter/5(Nout)
  Anti-windup/1(Out1) -> Tsamp - Integral/1(U)
  Ground_extTs/1 -> Tsamp - Integral/2(Ts), Filter/6(Ts), Tsamp - Ngain/2(Ts)
  Tsamp - Integral/1(Out1) -> Integrator/1(U)
  Tracking Mode/1(Out1) -> Tracking Mode Sum/2(fromTR)
  Ground_I0/1 -> Integrator ICs/1(I0)
  Filter ICs/1(Out1) -> Filter/4(D0in)
  N Copy/1(Out1) -> Filter/3(N)
  D Gain/1(Out1) -> Filter/2(U)
  Ground_D0/1 -> Filter ICs/1(D0)
  Ground_Reset/1 -> Reset Signal/1(Reset)
  N Gain/1(Out1) -> Tsamp - Ngain/1(U), Sum/3(D), Sum Fdbk/3(fromD)
  postSat Signal/1(Out1) -> Anti-windup/2(postSat), Tracking Mode/1(uout)
  preSat Signal/1(Out1) -> Anti-windup/1(preSat)
  Saturation Fdbk/1(Out1) -> postSat Signal/1(feedback)
  P Copy/1(Out1) -> Anti-windup/3(P)
  Ground_TR/1 -> Tracking Mode/2(TR)
  Ground_N/1 -> N Copy/1(N Gain), N Gain/2(N Gain)
  Ideal P Gain Fdbk/1(Out1) -> preSat Signal/1(feedback), Saturation Fdbk/1(In1)
  Sum Fdbk/1(Out1) -> Ideal P Gain Fdbk/1(In1)
  I Gain/1(Out1) -> Tracking Mode Sum/1(fromIgain)
  Saturation/1(Out1) -> y/1, postSat Signal/2(forward)
  Filter/1(Y) -> N Gain/1(U)
  Ground_D/1 -> D Gain/2(D Gain)
  Ideal P Gain/1(Out1) -> Saturation/1(In1), preSat Signal/2(forward)
  u/1 -> External Derivative/1(err), Parallel P Gain/1(err), I Gain/1(err)
  Parallel P Gain/1(Out1) -> Sum/1(P), Sum Fdbk/1(fromP)
  Sum/1(Out1) -> Ideal P Gain/1(In1)
  Ground_P/1 -> Ideal P Gain Fdbk/2(P Gain), Ideal P Gain/2(P Gain), Parallel P Gain/2(P Gain), P Copy/1(P Gain)
  Tracking Mode Sum/1(preInt) -> Terminator_preInt/1, preInt Signal/1(preInt)
  Ground_I/1 -> I Gain/2(I Gain)
  Integrator ICs/1(Out1) -> Integrator/2(I0in)
  Integrator/2(out) -> Sum/2(I)
  Integrator/1(state) -> Sum Fdbk/2(fromState)
  Reset Signal/1(Out1) -> Filter/1(Reset), Integrator/3(Reset)

== system BMD_2_backup/FCS/filters/Subsystem/body2earth ==
  ax,ay,az : Inport
  orient_f : Inport  Port=2
  Constant : Constant  Value=[0 0 -g]  OutDataTypeStr=single
  Data Type Conversion3 : DataTypeConversion  OutDataTypeStr=double  SaturateOnIntegerOverflow=off  RndMeth=Floor
  Demux : Demux  Outputs=3
  Math Function : Math  Operator=transpose
  Matrix Multiply : Product  Multiplication=Matrix(*)  OutDataTypeStr=single
  Minus : Sum
  Mux : Mux  Inputs=3
  Rotation Angles to Direction Cosine Matrix : Angle2Dcm
      settings: AttributesFormatString=Rotation Order: %<rotationOrder>
  Scope : Scope  NumInputPorts=2
      settings: ActiveDisplayYMinimum=-12.048131823539734  ActiveDisplayYMaximum=10.333153605461121  DataLoggingVariableName=ScopeData53
  Out1 : Outport
  wires:
  Minus/1 -> Scope/2, Out1/1  "axayaz_earth"
  Rotation Angles to Direction Cosine Matrix/1 -> Matrix Multiply/1
  ax,ay,az/1 -> Matrix Multiply/2
  Matrix Multiply/1 -> Minus/1
  Data Type Conversion3/1 -> Rotation Angles to Direction Cosine Matrix/1
  orient_f/1 -> Scope/1, Demux/1  "roll, pitch,yaw"
  Mux/1 -> Data Type Conversion3/1  "yaw,pitch,roll"
  Demux/2 -> Mux/2
  Demux/3 -> Mux/1
  Demux/1 -> Mux/3
  Constant/1 -> Minus/2

== system BMD_2_backup/FCS/filters/Subsystem/x,y,z,dy,dy,dz ==
  ax,ay,az_earth : Inport
  pressure_f : Inport  Port=2
  GPS_s : Inport  Port=3
  Demux : Demux  Outputs=3
  Mux : Mux  Inputs=3
  Mux1 : Mux  Inputs=3
  Mux2 : Mux  Inputs=2
  x.y.dx.dy : Subsystem
  z,dz : Subsystem
  x,y,z : Outport
  dx,dy,dz : Outport  Port=2
  wires:
  Mux/1 -> x,y,z/1
  ax,ay,az_earth/1 -> Demux/1
  Demux/3 -> z,dz/1(az)
  pressure_f/1 -> z,dz/2(alt)
  Mux1/1 -> dx,dy,dz/1
  x.y.dx.dy/1(dx) -> Mux1/1
  x.y.dx.dy/2(dy) -> Mux1/2
  x.y.dx.dy/3(x) -> Mux/1
  x.y.dx.dy/4(y) -> Mux/2
  z,dz/1(z) -> Mux/3
  z,dz/2(dz) -> Mux1/3
  GPS_s/1 -> x.y.dx.dy/1(GPS_s)
  Demux/1 -> Mux2/1
  Demux/2 -> Mux2/2
  Mux2/1 -> x.y.dx.dy/2(axay)
